simulink model "nav3"  (R2020a)
settings: Solver=FixedStepAuto  StartTime=0.0  StopTime=inf  RelTol=1e-3
model workspace (MAT data in the model file):
  SL_ROS_VariableLengthArrays_MaxSizes : object (value not decoded)
values from neighbouring files (symbols this model uses):
  map = binaryOccupancyMap(logicalMap, 1/0.05)    [exampleHelperVisualizeExecuteRobots.m]
undefined symbols (not defined in the file or in its folder): Angular, Data, Data_SL_Info, gray, Linear
libraries: robotlib x43, simulink x1
(part 2 of 2)

== matlab function nav3/Perception_Subsystem/SLAM_Subsystem/Live_Pose_Parser/World to Robot Transform ==
  data: pose input; robotPose output; W2ORTransform input; L2RTransform input
function robotPose = fcn(pose, W2ORTransform, L2RTransform)
    
    % W2LOTransform 
    W2LOTransform = W2ORTransform/(L2RTransform); 
    
    %LO2 Transform 
    LO2LTransform = [cos(pose(3,1)), -sin(pose(3,1)), pose(1,1);
                    sin(pose(3,1)), cos(pose(3,1)), pose(2,1);
                    0,              0,              1];

    % Calculate W2R = W2LO * LO2L * L2R
    W2RTransform = W2LOTransform*LO2LTransform*L2RTransform; 
    
    % Create 3D Rotation matrix
    rotm = [W2RTransform(1,1), W2RTransform(1,2), 0;
            W2RTransform(2,1), W2RTransform(2,2), 0; 
            0                , 0                , 1;]; 
    
    % Extract axis angle
    quat = rotm2quat(rotm);
    heading = quat2eul(quat); 
    
robotPose = [W2RTransform(1,3); W2RTransform(2,3); heading(1,1)];

== matlab function nav3/Perception_Subsystem/SLAM_Subsystem/Map_2_Image ==
  data: map input; image output size=[1000,1000]
function image = fcn(map)

image = imcomplement(flipud(map));

== matlab function nav3/Perception_Subsystem/IMU_Subsystem/Live_Pose_Parser/Quaternion_2_Euler ==
  data: x input; theta output; y input; z input; w input
function theta = fcn(x, y, z, w)

    euler = quat2eul([x, y, z, w]); 
    
    if sum(isnan(euler)) == 3
        
        euler = ([pi, 0, 0]);
        
    end 
    
theta = euler(1,3);

== matlab function nav3/Perception_Subsystem/SLAM_Subsystem/Live_Pose_Parser/Quaternion_2_Euler ==
  data: x input; theta output; y input; z input; w input
function theta = fcn(x, y, z, w)

    euler = quat2eul([x, y, z, w]); 
    
    if sum(isnan(euler)) == 3
        
        euler = ([pi, 0, 0]);
        
    end 
    
theta = euler(1,3);

== matlab function nav3/Parameter_Server_Subsystem/Robot_Parameters/MATLAB Function ==
  data: Lidar2RobotX input; Lidar2Robot output; Lidar2RobotY input; Lidar2RobotTheta input
function Lidar2Robot = fcn(Lidar2RobotX, Lidar2RobotY, Lidar2RobotTheta)
    
    Lidar2Robot = [cos(Lidar2RobotTheta), -sin(Lidar2RobotTheta), Lidar2RobotX;
                   sin(Lidar2RobotTheta), cos(Lidar2RobotTheta), Lidar2RobotY; 
                   0, 0, 1;];

== matlab function nav3/Parameter_Server_Subsystem/Experiment_Parameters/MATLAB Function ==
  data: initialPose input; World2RobotOdom output
function World2RobotOdom = fcn(initialPose)

    initialPoseX = initialPose(1,1); 
    initialPoseY = initialPose(2,1); 
    initialPoseTheta = initialPose(3,1); 

    World2RobotOdom = [cos(initialPoseTheta), -sin(initialPoseTheta), initialPoseX; 
                    sin(initialPoseTheta), cos(initialPoseTheta), initialPoseY; 
                    0            , 0            , 1];

== matlab function nav3/Perception_Subsystem/IMU_Subsystem/Live_Pose_Parser/TrueNorthToIMU1 ==
  data: orientation input; heading output; trueNorthAngle input
function heading = fcn(orientation, trueNorthAngle)


    % After testing 
    heading = orientation + trueNorthAngle; 
    
    % Ensure it is wrapped. 
    if heading >= pi 
        heading = heading - 2*pi; 
    elseif heading < -pi
        heading = heading + 2*pi; 
    end

== matlab function nav3/Perception_Subsystem/Camera_Subsystem/MATLAB Function ==
  data: image input; y output
function y = fcn(image)
    
    tagFamily = ['tag36h11']; 
    
    [id,loc,detectedFamily] = readAprilTag(image,tagFamily);
    
y = I;

== matlab function nav3/Perception_Subsystem/IMU_Subsystem/Live_Pose_Parser/TrueNorthToIMU ==
  data: orientation input; heading output
function heading = fcn(orientation)


    % After testing 
    heading = orientation + 1.99; 
    
    % Ensure it is wrapped. 
    if heading >= pi 
        heading = heading - 2*pi; 
    elseif heading < -pi
        heading = heading + 2*pi; 
    end

== matlab function nav3/Perception_Subsystem/IMU_Subsystem/Live_Pose_Parser/IMUToGround ==
  data: orientation input; heading output; trueNorthAngle input; initialPose input
function heading = fcn(orientation, trueNorthAngle, initialPose)

    % After testing 
    heading = orientation - trueNorthAngle + initialPose(3,1) ; 
    
    % Ensure it is wrapped. 
    if heading >= pi 
        heading = heading - 2*pi; 
    elseif heading < -pi
        heading = heading + 2*pi; 
    end

== matlab function nav3/Control_Subsystem/State_Machine/PID/Calculate_Error ==
  data: goalHeading input; currentHeading input; error output
function error = fcn(goalHeading, currentHeading)
    
    % Calculate basic error
    error = goalHeading - currentHeading;
    
    % Calculate angle wrap
    if error < -pi
        error = error + 2*pi;
    elseif error > pi
        error = (error - 2*pi);
    end

== matlab function nav3/Control_Subsystem/State_Machine/PID/Normalise_Heading ==
  data: headingAngle input; bearingAngle output
function bearingAngle = fcn(headingAngle)
 
    if headingAngle < 0
        headingAngle = pi + (pi - abs(headingAngle)); 
    end

bearingAngle = headingAngle;

== matlab function nav3/Control_Subsystem/State_Machine/PID/Normalise_Goal_Heading ==
  data: headingAngle input; bearingAngle output
function bearingAngle = fcn(headingAngle)
 
    if headingAngle < 0
        headingAngle = pi + (pi - abs(headingAngle)); 
    end

bearingAngle = headingAngle;
